simulink library "drones"  (R2015b)
settings: Solver=ode45  StartTime=0.0  StopTime=10.0  RelTol=1e-3
undefined symbols (not defined in the file or in its folder): C_trainee, mtot, Mw, Pw, rho
undefined symbols (not defined in the file): aero, drone, Imoteur, motor
settings Model: Creator=f.defay  LastModifiedBy=corentin
settings DataIOCC: SaveFormat=StructureWithTime
settings HardwareCC: ProdWordSize=32  ProdHWDeviceType=Specified

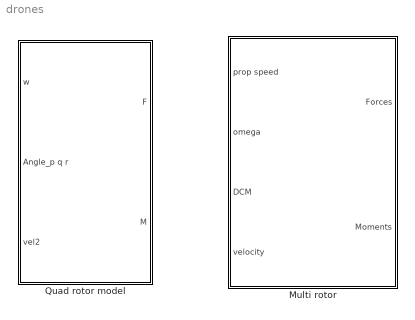
== system drones ==
  Multi rotor : Subsystem  mask{thrust_factor=Pw, torque_coef=Mw, density=rho, drag_coef=C_trainee(1)*3, rotor_inertia=Imoteur(1,1), prop_diameter=0.2, total_mass=mtot, aircraft_diameter=0.5, aircraft_type=1}
      mask prompts: thrust_factor "Thrust factor between w² and thrust"; torque_coef "Torque coefficient betwwen w² and torque"; density "Air density"; drag_coef "linear drag coefficient"; rotor_inertia "rotor inertia"; prop_diameter "propeller diameter"; total_mass "total mass"; aircraft_diameter "aircraft diameter"; aircraft_type "aircraft type: 4 rotors X (1), 4 rotors +(2), 6 rotors X (3)"
      mask TypeOptions aircraft_type: 1 | 2 | 3
  Quad rotor model : Subsystem  mask{Pw=motor.Pw, L=drone.lenght_arm, Mw=motor.Mw, mtot=drone.mtot, rho=aero.rho, S_drag_uvw=aero.S_trainee_uvw, C_drag=aero.C_trainee, g=aero.g, C_trainee=0, S_trainee_pqr=0}
      mask prompts: Pw "Thrust factor"; L "Length of the arm"; Mw "Torque coefficient"; mtot "Total mass"; rho "Air density"; S_drag_uvw "Drag Surface"; C_drag "Drag coefficient"; g "Gravity constant"; C_trainee "rotationnal drag coef"; S_trainee_pqr "rotationnal drag surface"

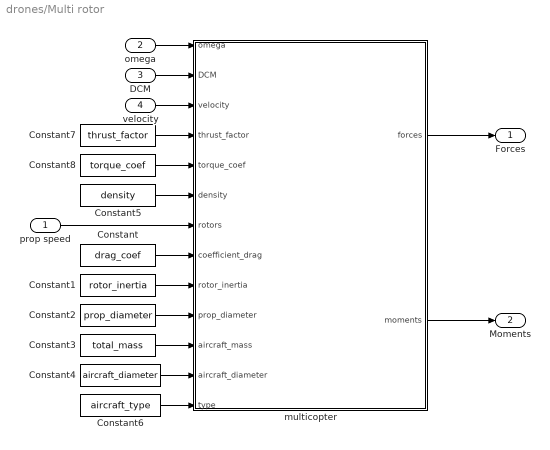
== system drones/Multi rotor ==
  prop speed : Inport
  omega : Inport  Port=2
  DCM : Inport  Port=3
  velocity : Inport  Port=4
  Constant : Constant  Value=drag_coef
  Constant1 : Constant  Value=rotor_inertia
  Constant2 : Constant  Value=prop_diameter
  Constant3 : Constant  Value=total_mass
  Constant4 : Constant  Value=aircraft_diameter
  Constant5 : Constant  Value=density
  Constant6 : Constant  Value=aircraft_type
  Constant7 : Constant  Value=thrust_factor
  Constant8 : Constant  Value=torque_coef
  multicopter : MATLAB Function  TreatAsAtomicUnit=on
  Forces : Outport
  Moments : Outport  Port=2
  wires:
  velocity/1 -> multicopter/3(velocity)
  prop speed/1 -> multicopter/7(rotors)
  Constant4/1 -> multicopter/12(aircraft_diameter)
  Constant5/1 -> multicopter/6(density)
  Constant3/1 -> multicopter/11(aircraft_mass)
  Constant2/1 -> multicopter/10(prop_diameter)
  multicopter/1(forces) -> Forces/1
  omega/1 -> multicopter/1(omega)
  DCM/1 -> multicopter/2(DCM)
  multicopter/2(moments) -> Moments/1
  Constant1/1 -> multicopter/9(rotor_inertia)
  Constant/1 -> multicopter/8(coefficient_drag)
  Constant6/1 -> multicopter/13(type)
  Constant7/1 -> multicopter/4(thrust_factor)
  Constant8/1 -> multicopter/5(torque_coef)

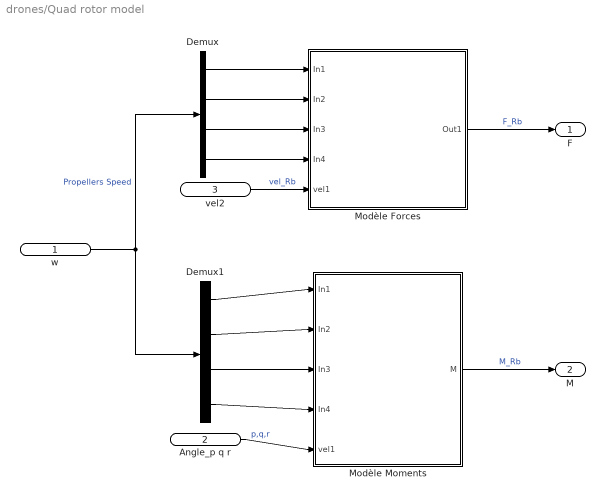
== system drones/Quad rotor model ==
  w : Inport
  Angle_p q r : Inport  Port=2
  vel2 : Inport  Port=3
  Demux : Demux
  Demux1 : Demux
  Modèle Forces : Subsystem
  Modèle Moments : Subsystem
  F : Outport
  M : Outport  Port=2
  wires:
  Modèle Moments/1(M) -> M/1  "M_Rb"
  Modèle Forces/1(Out1) -> F/1  "F_Rb"
  Angle_p q r/1 -> Modèle Moments/5(vel1)  "p,q,r"
  vel2/1 -> Modèle Forces/5(vel1)  "vel_Rb"
  Demux1/3 -> Modèle Moments/3(In3)
  Demux1/4 -> Modèle Moments/4(In4)
  Demux1/2 -> Modèle Moments/2(In2)
  Demux1/1 -> Modèle Moments/1(In1)
  Demux/3 -> Modèle Forces/3(In3)
  Demux/2 -> Modèle Forces/2(In2)
  Demux/4 -> Modèle Forces/4(In4)
  Demux/1 -> Modèle Forces/1(In1)
  w/1 -> Demux1/1, Demux/1  "Propellers Speed"

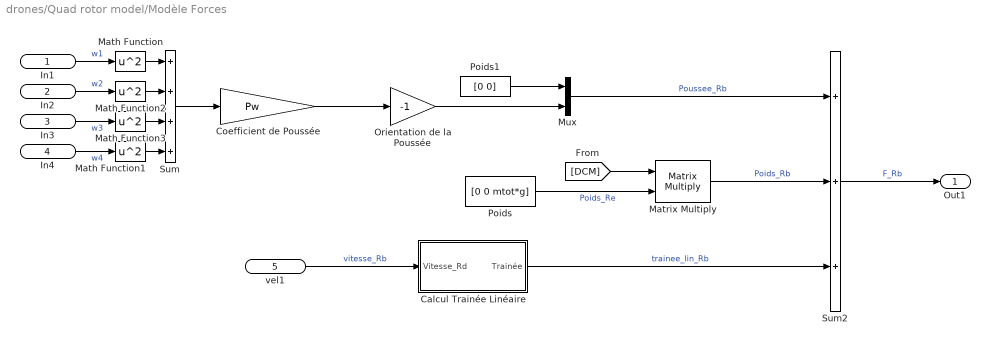
== system drones/Quad rotor model/Modèle Forces ==
  In1 : Inport
  In2 : Inport  Port=2
  In3 : Inport  Port=3
  In4 : Inport  Port=4
  vel1 : Inport  Port=5
  Calcul Trainée Linéaire : Subsystem
  Coefficient de Poussée : Gain  Gain=Pw
  Math Function{,1..3} (4 alike) : Math  Operator=square  SaturateOnIntegerOverflow=on
  Matrix Multiply : Product  Multiplication=Matrix(*)
  Mux : Mux  Inputs=2
  Orientation de la Poussée : Gain  Gain=-1
  Poids : Constant  Value=[0 0 mtot*g]  OutDataTypeStr=Inherit: Inherit via back propagation
  Poids1 : Constant  Value=[0 0]  OutDataTypeStr=Inherit: Inherit via back propagation
  Sum : Sum  Inputs=++++
  Sum2 : Sum  Inputs=+++
  Out1 : Outport
  wires:
  In4/1 -> Math Function1/1  "w4"
  In3/1 -> Math Function3/1  "w3"
  In2/1 -> Math Function2/1  "w2"
  In1/1 -> Math Function/1  "w1"
  Sum/1 -> Coefficient de Poussée/1
  Poids/1 -> Matrix Multiply/2  "Poids_Re"
  Coefficient de Poussée/1 -> Orientation de la Poussée/1
  Poids1/1 -> Mux/1
  Mux/1 -> Sum2/1  "Poussee_Rb"
  Sum2/1 -> Out1/1  "F_Rb"
  [DCM] -> Matrix Multiply/1
  Matrix Multiply/1 -> Sum2/2  "Poids_Rb"
  vel1/1 -> Calcul Trainée Linéaire/1(Vitesse_Rd)  "vitesse_Rb"
  Calcul Trainée Linéaire/1(Trainée) -> Sum2/3  "trainee_lin_Rb"
  Orientation de la Poussée/1 -> Mux/2
  Math Function3/1 -> Sum/3
  Math Function/1 -> Sum/1
  Math Function1/1 -> Sum/4
  Math Function2/1 -> Sum/2

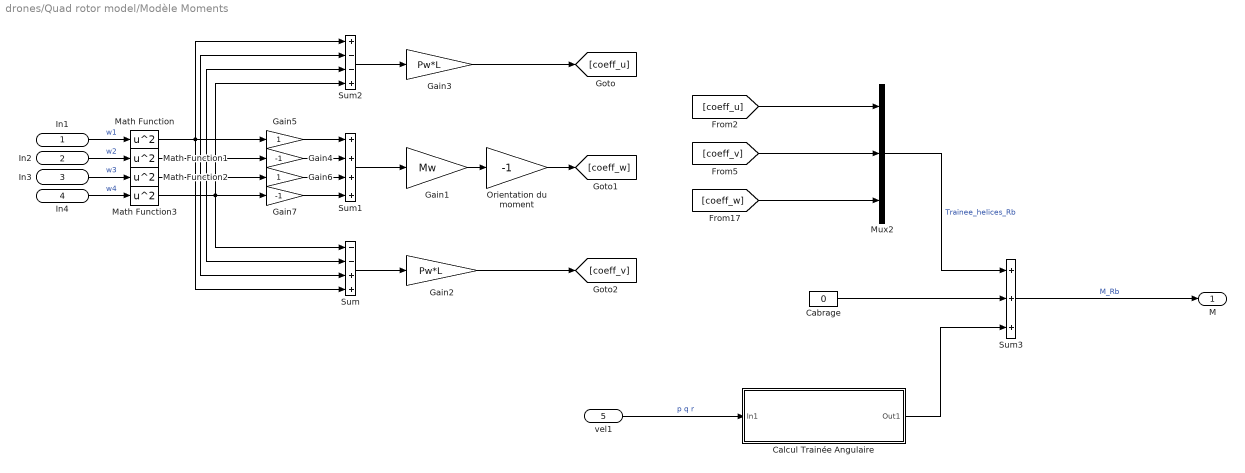
== system drones/Quad rotor model/Modèle Moments ==
  In1 : Inport
  In2 : Inport  Port=2
  In3 : Inport  Port=3
  In4 : Inport  Port=4
  vel1 : Inport  Port=5
  Cabrage : Constant  Value=0
  Calcul Trainée Angulaire : Subsystem
  Gain1 : Gain  Gain=Mw
  Gain2 : Gain  Gain=Pw*L
  Gain3 : Gain  Gain=Pw*L
  Gain4 : Gain  Gain=-1
  Gain5 : Gain
  Gain6 : Gain
  Gain7 : Gain  Gain=-1
  Math Function{,1..3} (4 alike) : Math  Operator=square  SaturateOnIntegerOverflow=on
  Mux2 : Mux  Inputs=3
  Orientation du moment : Gain  Gain=-1
  Sum : Sum  Inputs=--++
  Sum1 : Sum  Inputs=++++
  Sum2 : Sum  Inputs=+--+
  Sum3 : Sum  Inputs=+++
  M : Outport
  wires:
  In1/1 -> Math Function/1  "w1"
  In2/1 -> Math Function1/1  "w2"
  In4/1 -> Math Function3/1  "w4"
  In3/1 -> Math Function2/1  "w3"
  Sum2/1 -> Gain3/1
  Sum/1 -> Gain2/1
  Sum1/1 -> Gain1/1
  Gain1/1 -> Orientation du moment/1
  Gain4/1 -> Sum1/2
  Gain7/1 -> Sum1/4
  [coeff_w] -> Mux2/3
  Sum3/1 -> M/1  "M_Rb"
  Mux2/1 -> Sum3/1  "Trainee_helices_Rb"
  vel1/1 -> Calcul Trainée Angulaire/1(In1)  "p q r"
  Calcul Trainée Angulaire/1(Out1) -> Sum3/3
  Gain2/1 -> [coeff_v]
  Gain3/1 -> [coeff_u]
  [coeff_v] -> Mux2/2
  [coeff_u] -> Mux2/1
  Gain5/1 -> Sum1/1
  Gain6/1 -> Sum1/3
  Cabrage/1 -> Sum3/2
  Orientation du moment/1 -> [coeff_w]
  Math Function/1 -> Gain5/1, Sum/4, Sum2/1
  Math Function1/1 -> Gain4/1, Sum/3, Sum2/2
  Math Function2/1 -> Sum/2, Gain6/1, Sum2/3
  Math Function3/1 -> Gain7/1, Sum/1, Sum2/4

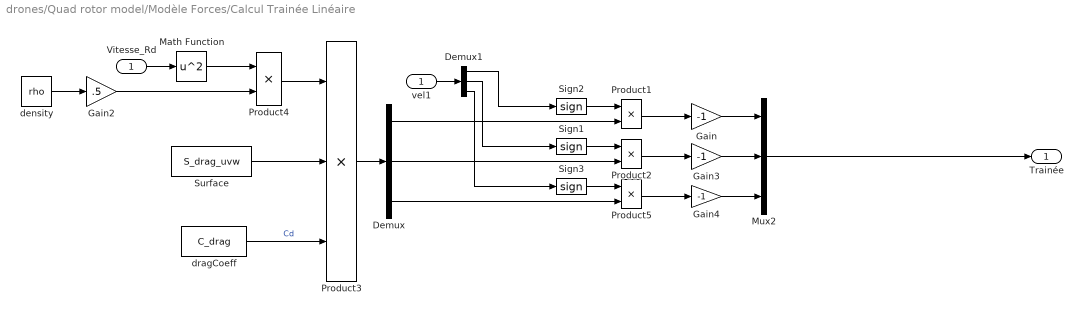
== system drones/Quad rotor model/Modèle Forces/Calcul Trainée Linéaire ==
  Vitesse_Rd : Inport
  Demux : Demux  Outputs=3
  Demux1 : Demux  Outputs=3
  Gain : Gain  Gain=-1
  Gain2 : Gain  Gain=.5
  Gain3 : Gain  Gain=-1
  Gain4 : Gain  Gain=-1
  Math Function : Math  Operator=square  SaturateOnIntegerOverflow=on
  Mux2 : Mux  Inputs=3
  Product{1..2,4..5} (4 alike) : Product  RndMeth=Zero
  Product3 : Product  Inputs=3  RndMeth=Zero
  Sign1 : Signum
  Sign2 : Signum
  Sign3 : Signum
  Surface : Constant  Value=S_drag_uvw  SampleTime=0
  density : Constant  Value=rho  SampleTime=0
  dragCoeff : Constant  Value=C_drag  SampleTime=0
  vel1 : InportShadow
  Trainée : Outport
  wires:
  Product3/1 -> Demux/1
  Gain4/1 -> Mux2/3
  Gain3/1 -> Mux2/2
  Gain/1 -> Mux2/1
  Demux/3 -> Product5/2
  Demux/2 -> Product2/2
  Demux/1 -> Product1/2
  Sign3/1 -> Product5/1
  Sign1/1 -> Product2/1
  Sign2/1 -> Product1/1
  Demux1/3 -> Sign3/1
  Demux1/2 -> Sign1/1
  Demux1/1 -> Sign2/1
  vel1/1 -> Demux1/1
  Product1/1 -> Gain/1
  Product2/1 -> Gain3/1
  Product5/1 -> Gain4/1
  Mux2/1 -> Trainée/1
  density/1 -> Gain2/1
  Surface/1 -> Product3/2
  dragCoeff/1 -> Product3/3  "Cd"
  Vitesse_Rd/1 -> Math Function/1
  Product4/1 -> Product3/1
  Math Function/1 -> Product4/1
  Gain2/1 -> Product4/2

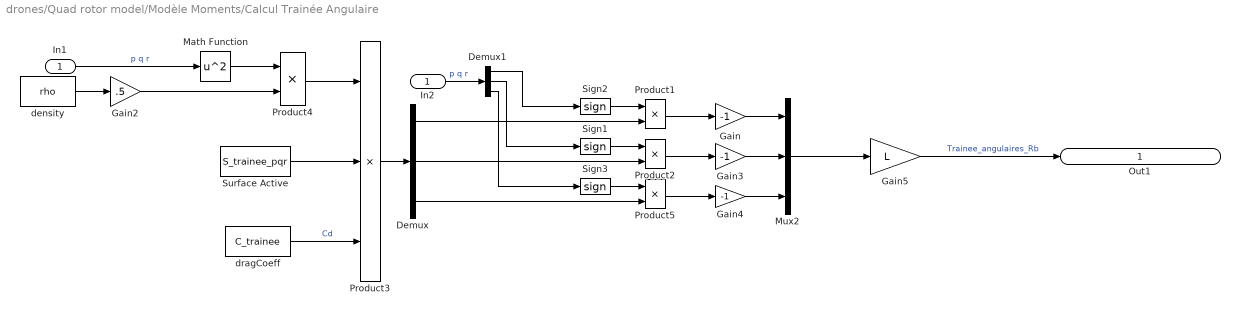
== system drones/Quad rotor model/Modèle Moments/Calcul Trainée Angulaire ==
  In1 : Inport
  Demux : Demux  Outputs=3
  Demux1 : Demux  Outputs=3
  Gain : Gain  Gain=-1
  Gain2 : Gain  Gain=.5
  Gain3 : Gain  Gain=-1
  Gain4 : Gain  Gain=-1
  Gain5 : Gain  Gain=L
  In2 : InportShadow
  Math Function : Math  Operator=square  SaturateOnIntegerOverflow=on
  Mux2 : Mux  Inputs=3
  Product{1..2,4..5} (4 alike) : Product  RndMeth=Zero
  Product3 : Product  Inputs=3  RndMeth=Zero
  Sign1 : Signum
  Sign2 : Signum
  Sign3 : Signum
  Surface Active : Constant  Value=S_trainee_pqr  SampleTime=0
  density : Constant  Value=rho  SampleTime=0
  dragCoeff : Constant  Value=C_trainee  SampleTime=0
  Out1 : Outport
  wires:
  Mux2/1 -> Gain5/1
  Gain5/1 -> Out1/1  "Trainee_angulaires_Rb"
  In1/1 -> Math Function/1  "p q r"
  Gain2/1 -> Product4/2
  Product4/1 -> Product3/1
  dragCoeff/1 -> Product3/3  "Cd"
  density/1 -> Gain2/1
  Product5/1 -> Gain4/1
  Product2/1 -> Gain3/1
  Product1/1 -> Gain/1
  In2/1 -> Demux1/1  "p q r"
  Demux1/1 -> Sign2/1
  Demux1/2 -> Sign1/1
  Demux1/3 -> Sign3/1
  Sign2/1 -> Product1/1
  Sign1/1 -> Product2/1
  Sign3/1 -> Product5/1
  Demux/1 -> Product1/2
  Demux/2 -> Product2/2
  Demux/3 -> Product5/2
  Gain/1 -> Mux2/1
  Gain3/1 -> Mux2/2
  Gain4/1 -> Mux2/3
  Math Function/1 -> Product4/1
  Product3/1 -> Demux/1
  Surface Active/1 -> Product3/2

== matlab function drones/Multi rotor/multicopter ==
  data: omega input; DCM input; velocity input; thrust_factor input; torque_coef input; density input; rotors input; forces output; moments output; coefficient_drag input; rotor_inertia input; prop_diameter input; aircraft_mass input; aircraft_diameter input; type input
function [forces, moments] = multicopter(omega, DCM, velocity, thrust_factor,torque_coef,density, rotors,coefficient_drag,rotor_inertia,prop_diameter,aircraft_mass,aircraft_diameter,type)

%================================Constants=================================

%coefficient_drag = 15;              % coefficient of drag
%rotor_inertia = 0.0000025;          % rotor inertia                         (kg m^2)
%prop_diameter = 0.1397;             % diameter of the propellor             (meters)                                 
%aircraft_mass = 0.26;               % aircraft mass                         (kg)                                        
%aircraft_diameter = 0.25;           % motor to motor distance               (meters)                                      

%==============================Actuator Mixer==============================

% [x(roll), y(pitch), z(yaw)]
MIX = [  0   0   0   ;      % QUAD [X]
         0   0   0   ;
         0   0   0   ;
         0   0   0   ;
         0   0   0   ;
         0   0   0   ;
         0   0   0   ;
         0   0   0   ];
     
switch type
    case 1
        
MIX = [  1   1  -1   ;      % QUAD [X]
        -1   1   1   ;
        -1  -1  -1   ;
         1  -1   1   ;
         0   0   0   ;
         0   0   0   ;
         0   0   0   ;
         0   0   0   ];

    case 2
MIX = [  0   1  -1   ;      % QUAD [+]
        -1   0   1   ;
         0  -1  -1   ;
         1   0   1   ;
         0   0   0   ;
         0   0   0   ;
         0   0   0   ;
         0   0   0   ];
    case 3
MIX = [  1   1  -1   ;      % HEX [X]
        -1   1   1   ;
        -1   0  -1   ;
        -1  -1   1   ;
         1  -1  -1   ;
         1   0   1   ;
         0   0   0   ;
         0   0   0   ];

end
%==================================Forces================================== 

a = [   aircraft_diameter^2 / 10                        ;...                % body cross sectional area (X)
        aircraft_diameter^2 / 10                        ;...                % body cross sectional area (Y)
        sum(abs(MIX(:, 3))) * pi/4 * prop_diameter^2    ];                  % body cross sectional area (Z)
    
gravity = aircraft_mass .* (DCM * [0; 0; 9.81]);                            % gravitational force
drag = -velocity .* coefficient_drag .* density .* a;                       % drag force

%--------------------------------Thrust Model------------------------------
thrust = abs(MIX(:, 3)) .* thrust_factor .* rotors .* rotors;                              % rotor thrust <==     
%--------------------------------------------------------------------------

forces = gravity + drag;
forces(3) = forces(3) - sum(thrust);

%==================================Moments=================================

mx = thrust .* MIX(:,1) .* (aircraft_diameter / 2)*sind(45);                % x moment
my = thrust .* MIX(:,2) .* (aircraft_diameter / 2)*sind(45);                % y moment

momentum_x = sum(abs(MIX(:, 3)) .* rotor_inertia .* rotors) * omega(1);     % x rotor momentum
momentum_y = sum(abs(MIX(:, 3)) .* rotor_inertia .* rotors) * omega(2);     % y rotor momentum
momentum_z = sum(MIX(:, 3) .* rotor_inertia .* rotors) * omega(3);          % z rotor momentum

%--------------------------------Torque Model------------------------------
mz = MIX(:,3) .* torque_coef .* rotors .* rotors;                                        % rotor torque <==
%--------------------------------------------------------------------------

moments = [sum(mx); sum(my); sum(mz)] - [momentum_x; momentum_y; momentum_z];

%==========================================================================
